simulink model "nonlinear_linear_comparison"  (R2017a)
settings: Solver=ode4  StartTime=0.0  StopTime=inf  FixedStep=0.1  RelTol=1e-3
values from neighbouring files (symbols this model uses):
  psi_op = pi/2    (= 1.57079632679)    [initialization_file.m]
  theta_op = -10*pi/180    (= -0.174532925199)    [initialization_file.m]
  Vmp_op = (Kyy*m_heli*g*cos(theta_op)*l_cm)/(Kyy*Kpp-Kyp*Kpy)    [initialization_file.m]
  Vmy_op = Kyp*Vmp_op/Kyy    [initialization_file.m]
  w_psi_op = 0    [initialization_file.m]
  w_theta_op = 0    [initialization_file.m]
libraries: realtime_pacer_lib x1
settings Model: SnapshotBufferSize=1000  SnapshotInterval=1000  Creator=Roshan  LastModifiedBy=rosha
settings RTWCC: SystemTargetFile=sldrt.tlc  TemplateMakefile=sldrt.tmf  Description=Simulink Desktop Real-Time  RTWCompilerOptimization=on
settings CodeAppCC: MaxIdLength=95
settings SimulinkDesktopRealTimeCC: TargetPreCompLibLocation=C:\Program Files\MATLAB\R2017a\toolbox\sldrt\lib\win64  SupportVariableSizeSignals=off

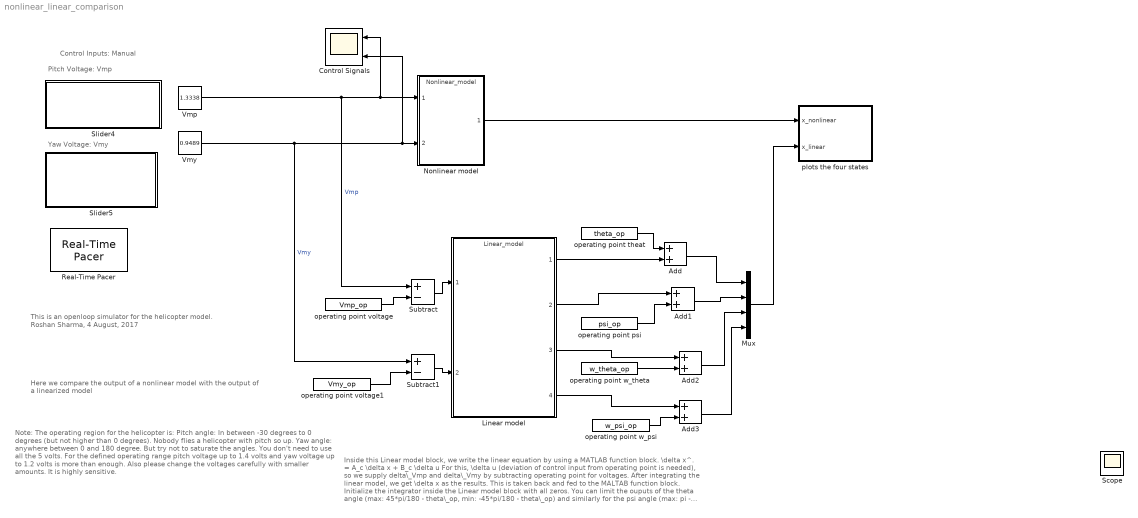
== system nonlinear_linear_comparison ==
  note: Inside this Linear model block, we write the linear equation by using a MATLAB function block.
      |
      | \delta x^.  = A_c \delta x + B_c \delta u
      |
      | For this, \delta u (deviation of control input from operating point is needed), so we supply delta\_Vmp and delta\_Vmy by
      | subtracting operating point for voltages.
      |
      | After integrating the linear model, we get \delta x as the results. This is taken back and fed to the MALTAB function block.
      | Initialize the integrator inside the Linear model block with all zeros. You can limit the ouputs of the
      | theta angle (max: 45*pi/180 - theta\_op, min:  -45*pi/180 - theta\_op) and similarly for the psi angle (max: pi - psi\_op, min:  0 - psi\_op).
      | You do not need to limit the output for the velocities.
      | Out from the linear model block, we obtain \delta x. To obtain x from \delta x, we add the operating point for states.
      |
      | To use variables loaded in the workspace in Simulink (for e.g. A_c, B_c etc.), make use of constant blocks. Instead of typing number
      | to a constant block, you can write down the name of the variable.  You can pass variables such as A_c as inputs to the MATLAB  function
      | block by connecting the constant block with defined variable names to the input of the MATLAB funciton block.
  note: Note: The operating region for the helicopter is:
      | Pitch angle: In between -30 degrees to 0 degrees (but not higher than
      | 0 degrees). Nobody flies a helicopter with pitch so up.
      | Yaw angle: anywhere between 0 and 180 degree.
      |
      | But try not to saturate the angles.
      |
      | You don't need to use all the 5 volts. For the defined operating range
      | pitch voltage up to 1.4 volts and yaw voltage up to 1.2 volts
      | is more than enough. Also please change the voltages carefully
      | with smaller amounts. It is highly sensitive.
  note: Here we compare the output of a nonlinear model with the output of a linearized model
  note: Control Inputs: Manual
  note: This is an openloop simulator
      | for the helicopter model.
      | Roshan Sharma, 4 August, 2017
  note: Pitch Voltage: Vmp
  note: Yaw Voltage: Vmy
  Add{,1..3} (4 alike) : Sum
  Control Signals : Scope  NumInputPorts=2
  Linear model : ModelReference  ModelNameDialog=Linear_model  ModelReferenceVersion=1.1040  CopyOfModelProtected=on
  Mux : Mux
  Nonlinear model : ModelReference  ModelNameDialog=Nonlinear_model  ModelReferenceVersion=1.1017  CopyOfModelProtected=on
  Real-Time Pacer : realtime_pacer_lib/Real-Time Pacer  simTimePerRealTime=1
  Slider4 : Subsystem  DialogController=hmiCreateDDGDialog  IsWebBlock=on  mask(MWDashboardBlock){webBlockId=d7fa2b72-57f0-4581-a642-3c1b7216c1b6, webBlockType=slider, ShowInLibBrowser=on, ShowInitialText=on, HMISrcModelName=nonlinear_linear_comparison}
      mask prompts: webBlockId "WebBlock Id"; webBlockType "WebBlock Type"; HMISrcModelName "Source Model"
      mask help: SimulinkHMI:dialogs:SliderDialogDesc
      mask Help: helpview([docroot '/mapfiles/simulink.map'], 'hmi_slider')
      mask Display:
      | if strcmp(get_param(bdroot(gcb),'BlockDiagramType'), 'library')
      |     image([(matlabroot) '/toolbox/simulink/hmi/icons/Slider.png']);
      | end
  Slider5 : Subsystem  DialogController=hmiCreateDDGDialog  IsWebBlock=on  mask(MWDashboardBlock){webBlockId=2da1ea5c-a5f5-4938-b925-ee22b86d0a23, webBlockType=slider, ShowInLibBrowser=on, ShowInitialText=on, HMISrcModelName=nonlinear_linear_comparison}
      mask prompts: webBlockId "WebBlock Id"; webBlockType "WebBlock Type"; HMISrcModelName "Source Model"
      mask help: SimulinkHMI:dialogs:SliderDialogDesc
      mask Help: helpview([docroot '/mapfiles/simulink.map'], 'hmi_slider')
      mask Display:
      | if strcmp(get_param(bdroot(gcb),'BlockDiagramType'), 'library')
      |     image([(matlabroot) '/toolbox/simulink/hmi/icons/Slider.png']);
      | end
  Subtract : Sum  Inputs=+-
  Subtract1 : Sum  Inputs=+-
  Vmp : Constant  Value=1.3338
  Vmy : Constant  Value=0.9489
  operating point psi : Constant  Value=psi_op
  operating point theat : Constant  Value=theta_op
  operating point voltage : Constant  Value=Vmp_op
  operating point voltage1 : Constant  Value=Vmy_op
  operating point w_psi : Constant  Value=w_psi_op
  operating point w_theta : Constant  Value=w_theta_op
  plots the four states : Subsystem
  Scope : Scope
  wires:
  Vmp/1 -> Subtract/1, Nonlinear model/1, Control Signals/1  "Vmp"
  Vmy/1 -> Subtract1/1, Nonlinear model/2, Control Signals/2  "Vmy"
  Nonlinear model/1 -> plots the four states/1(x_nonlinear)
  Subtract/1 -> Linear model/1
  operating point voltage/1 -> Subtract/2
  Subtract1/1 -> Linear model/2
  operating point voltage1/1 -> Subtract1/2
  Linear model/1 -> Add/2
  operating point theat/1 -> Add/1
  Linear model/2 -> Add1/1
  operating point psi/1 -> Add1/2
  Linear model/3 -> Add2/1
  operating point w_theta/1 -> Add2/2
  Linear model/4 -> Add3/1
  Add/1 -> Mux/1
  Add1/1 -> Mux/2
  Add2/1 -> Mux/3
  Add3/1 -> Mux/4
  Mux/1 -> plots the four states/2(x_linear)
  operating point w_psi/1 -> Add3/2

== system nonlinear_linear_comparison/Slider4 ==

== system nonlinear_linear_comparison/Slider5 ==

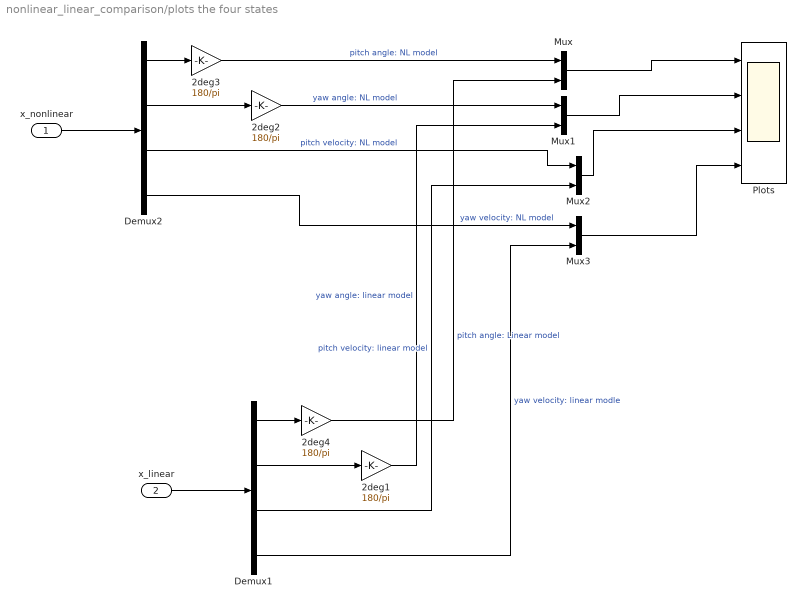
== system nonlinear_linear_comparison/plots the four states ==
  x_nonlinear : Inport
  x_linear : Inport  Port=2
  2deg{1..4} (4 alike) : Gain  Gain=180/pi
  Demux1 : Demux
  Demux2 : Demux
  Mux{,1..3} (4 alike) : Mux  Inputs=2
  Plots : Scope  NumInputPorts=4
  wires:
  x_nonlinear/1 -> Demux2/1
  Demux2/1 -> 2deg3/1
  Demux2/2 -> 2deg2/1
  2deg3/1 -> Mux/1  "pitch angle: NL model"
  2deg2/1 -> Mux1/1  "yaw angle: NL model"
  Demux2/3 -> Mux2/1  "pitch velocity: NL model"
  Demux2/4 -> Mux3/1  "yaw velocity: NL model"
  Demux1/4 -> Mux3/2  "yaw velocity: linear modle"
  x_linear/1 -> Demux1/1
  Demux1/1 -> 2deg4/1
  2deg1/1 -> Mux1/2  "yaw angle: linear model"
  2deg4/1 -> Mux/2  "pitch angle: Linear model"
  Demux1/2 -> 2deg1/1
  Demux1/3 -> Mux2/2  "pitch velocity: linear model"
  Mux/1 -> Plots/1
  Mux1/1 -> Plots/2
  Mux2/1 -> Plots/3
  Mux3/1 -> Plots/4
